simulink model "NewSignalGenerator"  (R2026a)
settings: Solver=VariableStepAuto  StopTime=5e-4
values from neighbouring files (symbols this model uses):
  ImTable = zeros(N,1)    [suggestion.m]
  RealTable = zeros(N,1)    [suggestion.m]
libraries: hdlsllib x1, dsphdlxfrm2 x1
settings Model: Creator=adams  LastModifiedBy=adams
settings OptimizationCC: ConditionallyExecuteInputs=off

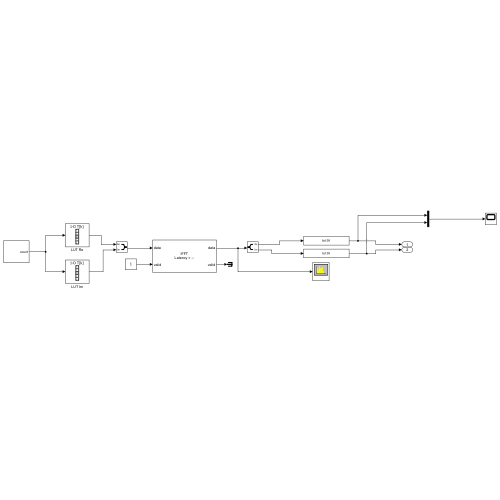
[thumbnail: Simulink's stored preview of the top-level diagram]
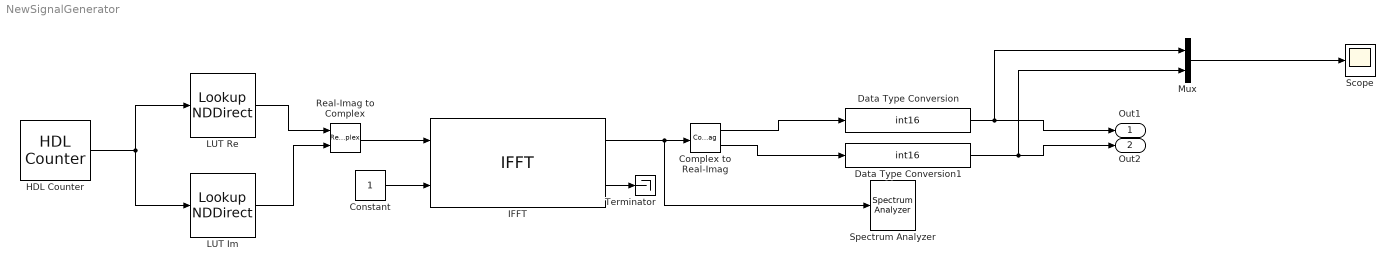
== system NewSignalGenerator ==
  Complex to Real-Imag : ComplexToRealImag
  Constant : Constant  OutDataTypeStr=boolean
  Data Type Conversion : DataTypeConversion  OutDataTypeStr=int16  SaturateOnIntegerOverflow=off  RndMeth=Floor
  Data Type Conversion1 : DataTypeConversion  OutDataTypeStr=int16  SaturateOnIntegerOverflow=off  RndMeth=Floor
  HDL Counter : hdlsllib/Sources/HDL Counter  CountType=Count limited  CountInit=0  CountStep=1  CountMax=511  CountFromType=Initial value  CountFrom=0  CountResetPort=off  CountLoadPort=off  CountEnbPort=off  CountDirPort=off  CountHitOutputPort=off  CountDataType=Unsigned  CountWordLen=9  CountFracLen=0  CountSampTime=4/614400000
  IFFT : dsphdlxfrm2/IFFT  Architecture=Streaming Radix 2^2  FFTLengthSource=Property  FFTLength=512  FFTLengthMax=1024  ComplexMultiplication=Use 4 multipliers and 2 adders  BitReversedOutput=off  BitReversedInput=off  Normalize=off  SimulateUsing=Code generation  RoundingMethod=Floor  ResetInputPort=off  StartOutputPort=off  EndOutputPort=off
  LUT Im : LookupNDDirect  NumberOfTableDimensions=1  Table=ImTable  TableDataTypeStr=fixdt(1,32,20)
  LUT Re : LookupNDDirect  NumberOfTableDimensions=1  Table=RealTable  TableDataTypeStr=fixdt(1,32,20)
  Mux : Mux  Inputs=2
  Real-Imag to Complex : RealImagToComplex
  Scope : Scope
      settings: ActiveDisplayYMinimum=-32234  ActiveDisplayYMaximum=31696
  Spectrum Analyzer : SpectrumAnalyzer  WindowPosition=[193.000000,171.000000,1086.000000,436.000000,]  ScopeFrameLocation=window  Method=Welch  RBWSource=Property  RBW=5000  WindowInvariantSamplesPerUpdate=on  FrequencySpan=Span and center frequency  Span=100000000  StartFrequency=-76800000  StopFrequency=76800000  Window=Hamming  YLimits=[-48.6742 112.0646]  SelectedToolstripTab=spectrumAnalyzerToolstrip.estimationTab
  Terminator : Terminator
  Out1 : Outport
  Out2 : Outport  Port=2
  wires:
  HDL Counter/1 -> LUT Im/1, LUT Re/1
  LUT Re/1 -> Real-Imag to Complex/1
  LUT Im/1 -> Real-Imag to Complex/2
  Real-Imag to Complex/1 -> IFFT/1
  Constant/1 -> IFFT/2
  IFFT/1 -> Spectrum Analyzer/1, Complex to Real-Imag/1
  Complex to Real-Imag/1 -> Data Type Conversion/1
  Complex to Real-Imag/2 -> Data Type Conversion1/1
  Data Type Conversion1/1 -> Mux/2, Out2/1
  Data Type Conversion/1 -> Mux/1, Out1/1
  Mux/1 -> Scope/1
  IFFT/2 -> Terminator/1
